simulink model "mcb_host_model_f28069m"  (R2025b)
settings: Solver=FixedStepDiscrete  StartTime=0.0  StopTime=inf  RelTol=1e-3  EnableMultiTasking=on
values from neighbouring files (symbols this model uses):
  PU_System = mcb.getPUSystemParameters(bldc,inverter)    [mcb_bldc_sixstep_f28069mLaunchPad_data.m]    (also in mcb_bldc_sixstep_f28379d_data.m = mcb.getPUSystemParameters(bldc, inverter))
  Ts = T_pwm    (= 5e-05)    [mcb_bldc_sixstep_f28069mLaunchPad_data.m]    (also in mcb_bldc_sixstep_f28379d_data.m = 3e-05)
libraries: instrumentseriallib x3
settings Model: Creator=The MathWorks, Inc.  LastModifiedBy=The MathWorks, Inc.
settings SolverCC: AlgebraicLoopSolver=TrustRegion  MaxZcPerStep=1.0
settings DataIOCC: LimitDataPoints=on  SaveFormat=Array  ReturnWorkspaceOutputs=off
settings OptimizationCC: ReuseModelBlockBuffer=off  LifeSpan=1  EfficientTunableParamExpr=on
settings DebuggingCC: UnderspecifiedInitializationDetection=Classic  MergeDetectMultiDrivingBlocksExec=none  SolverPrmCheckMsg=warning  ParameterPrecisionLossMsg=none  UnconnectedInputMsg=warning  UnconnectedOutputMsg=warning  UnconnectedLineMsg=warning  AllowSymbolicDim=off  PregeneratedLibrarySubsystemCodeDiagnostic=none  SFUnexpectedBacktrackingDiag=warning  SFNoUnconditionalDefaultTransitionDiag=warning  SFExecutionAtInitializationDiag=none  ArithmeticOperatorsInVariantConditions=warning
settings HardwareCC: ProdBitPerPointer=32.0  ProdLargestAtomicFloat=None  ProdIntDivRoundTo=Undefined  ProdEndianess=Unspecified  ProdWordSize=32.0  ProdHWDeviceType=32-bit Generic
settings ModelReferenceCC: EnableRefExpFcnMdlSchedulingChecks=on  PropagateSignalLabelsOutOfModel=off
settings SFSimCC: SimUseLocalCustomCode=off  MATLABDynamicMemAlloc=off
settings RTWCC: SystemTargetFile=ert.tlc  TemplateMakefile=ert_default_tmf  GenerateReport=on  RTWUseLocalCustomCode=off  IncludeHyperlinkInReport=on  LaunchReport=on  GenerateTraceInfo=on  GenerateTraceReport=on  GenerateTraceReportSl=on  GenerateTraceReportSf=on  GenerateTraceReportEml=on  GPUComputeCapability=3.5  DLArmComputeVersion=19.05  Description=Real-Time Workshop Embedded Coder
settings CodeAppCC: IgnoreCustomStorageClasses=off  StateflowObjectComments=on  InternalIdentifier=Classic
settings ERTTargetCC: InlinedParameterPlacement=Hierarchical  ERTCustomFileTemplate=example_file_process.tlc  ConvertIfToSwitch=off  SuppressUnreachableDefaultCases=off  DynamicArrayContainerType=coder::array  MultiwordLength=2048.0  GenerateSampleERTMain=on
settings ConfigComp: CovMetricSettings=dw  CovSaveCumulativeToWorkspaceVar=on  CovSaveSingleToWorkspaceVar=on  CovExternalEMLEnable=off  CovSFcnEnable=off

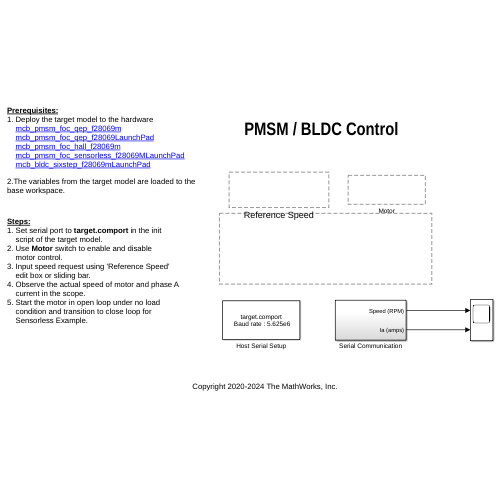
[thumbnail: Simulink's stored preview of the top-level diagram]
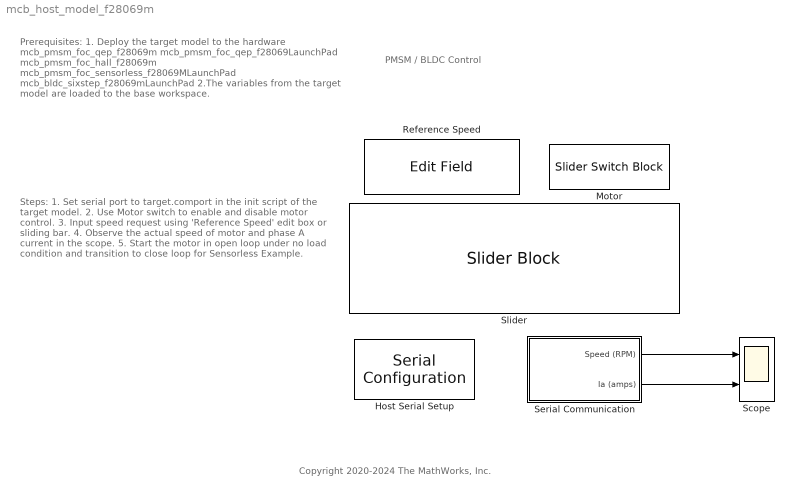
== system mcb_host_model_f28069m ==
  note: Copyright 2020-2024 The MathWorks, Inc.
  note: Steps:
      | 1. Set serial port to target.comport in the init
      | script of the target model.
      | 2. Use Motor switch to enable and disable
      | motor control.
      | 3. Input speed request using 'Reference Speed'
      | edit box or sliding bar.
      | 4. Observe the actual speed of motor and phase A
      | current in the scope.
      | 5. Start the motor in open loop under no load
      | condition and transition to close loop for
      | Sensorless Example.
  note: PMSM / BLDC Control
  note: Prerequisites:
      | 1. Deploy the target model to the hardware
      | mcb_pmsm_foc_qep_f28069m
      | mcb_pmsm_foc_qep_f28069LaunchPad
      | mcb_pmsm_foc_hall_f28069m
      | mcb_pmsm_foc_sensorless_f28069MLaunchPad
      | mcb_bldc_sixstep_f28069mLaunchPad
      |
      | 2.The variables from the target model are loaded to the base workspace.
  Host Serial Setup : instrumentseriallib/Serial Configuration  Priority=-99  PortSel=target.comport  Port=target.comport  ComPort=target.comport  BaudRate=5.625e6  DataBits=8  Parity=none  StopBits=1  ByteOrder=little-endian  FlowControl=none  Timeout=2  SimulateUsing=Interpreted execution  BlockInModel=on  aMode=5
      settings: LibrarySourceBlock=mcblib/Protection and Diagnostics/Host Serial Setup
  Motor : SliderSwitchBlock  LabelPosition=Hide
  Reference Speed : EditField  LabelPosition=Hide  ShowInitialText=on  Alignment=Center
  Scope : Scope  NumInputPorts=2
      settings: Title=Speed  ActiveDisplayYMinimum=-6000  ActiveDisplayYMaximum=6000  YLabel=Speed (RPM)
  Serial Communication : Subsystem
  Slider : SliderBlock  LabelPosition=Hide  ScaleMin=-6000  ScaleMax=6000
  wires:
  Serial Communication/1(Speed (RPM)) -> Scope/1
  Serial Communication/2(Ia (amps)) -> Scope/2

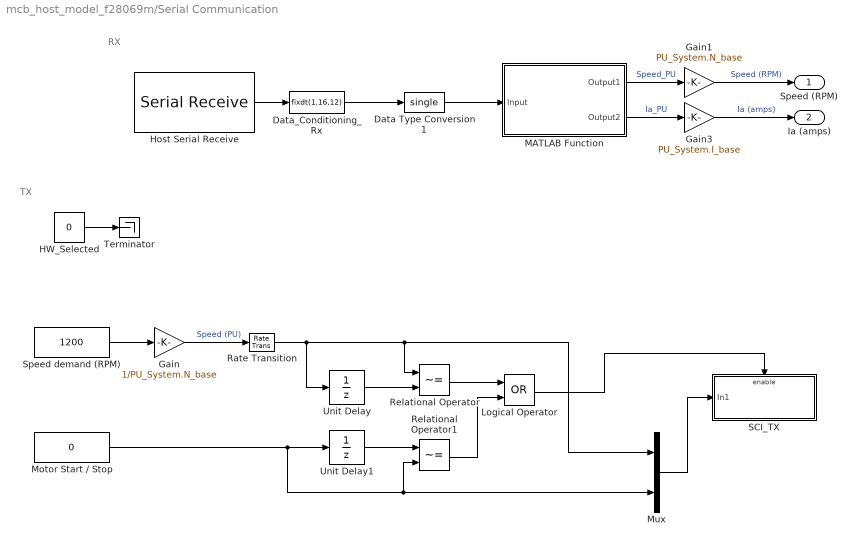
== system mcb_host_model_f28069m/Serial Communication ==
  note: RX
  note: TX
  Data Type Conversion1 : DataTypeConversion  OutDataTypeStr=single  RndMeth=Simplest  SaturateOnIntegerOverflow=off
  Data_Conditioning_Rx : DataTypeConversion  OutDataTypeStr=fixdt(1,16,12)  ConvertRealWorld=Stored Integer (SI)  RndMeth=Simplest  SaturateOnIntegerOverflow=off
  Gain : Gain  Gain=1/PU_System.N_base  RndMeth=Simplest  OutDataTypeStr=Inherit: Same as input
  Gain1 : Gain  Gain=PU_System.N_base  OutDataTypeStr=single  RndMeth=Simplest
  Gain3 : Gain  Gain=PU_System.I_base  OutDataTypeStr=single  RndMeth=Simplest
  HW_Selected : Constant  Value=0  OutDataTypeStr=uint8
  Host Serial Receive : instrumentseriallib/Serial Receive  PortSel=target.comport  Port=target.comport  ComPort=target.comport  DataType=uint16  SaveDataType=uint8  ToggleHeader=on  Header='SS'  ToggleDataSize=on  DataSize=[600 2]  ToggleTerminator=on  Terminator=Custom terminator  CustomTerminator='EE'  InputFormat=Row major  EnableBlockingMode=on  ActionDataUnavailable=Output last received value  ActionWhenDataUnavailable=Output last received value  CustomValue=0  SampleTime=600 * Ts  SimulateUsing=Interpreted execution  BlockInModel=on  aMode=5  LibraryInUse=instrumentlib
      settings: LibrarySourceBlock=mcblib/Protection and Diagnostics/Host Serial Receive
  Logical Operator : Logic  Operator=OR  AllPortsSameDT=off  OutDataTypeStr=boolean
  MATLAB Function : MATLAB Function  TreatAsAtomicUnit=on
  Motor Start / Stop : Constant  Value=0  VectorParams1D=off  OutDataTypeStr=single  SampleTime=0.03
  Mux : Mux  Inputs=2
  Rate Transition : RateTransition  OutPortSampleTime=0.03
  Relational Operator : RelationalOperator  Operator=~=  OutDataTypeStr=boolean  InputSameDT=off
  Relational Operator1 : RelationalOperator  Operator=~=  OutDataTypeStr=boolean  InputSameDT=off
  SCI_TX : Subsystem  TreatAsAtomicUnit=on
  Speed demand (RPM) : Constant  Value=1200  VectorParams1D=off  OutDataTypeStr=single  SampleTime=0.03
  Terminator : Terminator
  Unit Delay : UnitDelay  InitialCondition=0.5  SampleTime=-1  HasFrameUpgradeWarning=on
  Unit Delay1 : UnitDelay  SampleTime=-1  HasFrameUpgradeWarning=on
  Speed (RPM) : Outport
  Ia (amps) : Outport  Port=2
  wires:
  HW_Selected/1 -> Terminator/1
  Unit Delay1/1 -> Relational Operator1/1
  Relational Operator1/1 -> Logical Operator/2
  Unit Delay/1 -> Relational Operator/2
  Relational Operator/1 -> Logical Operator/1
  Gain/1 -> Rate Transition/1  "Speed (PU)"
  Speed demand (RPM)/1 -> Gain/1
  Mux/1 -> SCI_TX/1(In1)
  Rate Transition/1 -> Unit Delay/1, Mux/1, Relational Operator/1
  Logical Operator/1 -> SCI_TX/Enable
  Motor Start / Stop/1 -> Relational Operator1/2, Mux/2, Unit Delay1/1
  MATLAB Function/2(Output2) -> Gain3/1  "Ia_PU"
  Gain3/1 -> Ia (amps)/1  "Ia (amps)"
  Host Serial Receive/1 -> Data_Conditioning_Rx/1
  MATLAB Function/1(Output1) -> Gain1/1  "Speed_PU"
  Gain1/1 -> Speed (RPM)/1  "Speed (RPM)"
  Data_Conditioning_Rx/1 -> Data Type Conversion1/1
  Data Type Conversion1/1 -> MATLAB Function/1(Input)

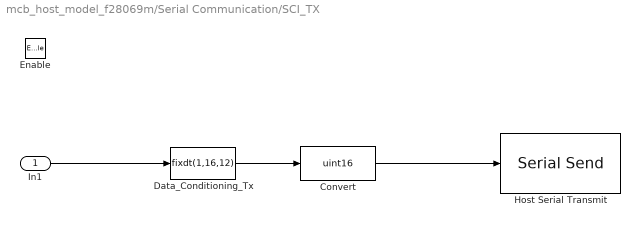
== system mcb_host_model_f28069m/Serial Communication/SCI_TX ==
  In1 : Inport
  Enable : EnablePort
  Convert : DataTypeConversion  OutDataTypeStr=uint16  ConvertRealWorld=Stored Integer (SI)  RndMeth=Simplest  SaturateOnIntegerOverflow=off
  Data_Conditioning_Tx : DataTypeConversion  OutDataTypeStr=fixdt(1,16,12)  RndMeth=Simplest  SaturateOnIntegerOverflow=off
  Host Serial Transmit : instrumentseriallib/Serial Send  PortSel=target.comport  Port=target.comport  ComPort=target.comport  Header=[]  Terminator=<none>  CustomTerminator=[]  EnableBlockingMode=off  SimulateUsing=Interpreted execution  BlockInModel=on  aMode=5
      settings: LibrarySourceBlock=mcblib/Protection and Diagnostics/Host Serial Transmit
  wires:
  Convert/1 -> Host Serial Transmit/1
  Data_Conditioning_Tx/1 -> Convert/1
  In1/1 -> Data_Conditioning_Tx/1

== matlab function mcb_host_model_f28069m/Serial Communication/MATLAB Function ==
  data: Output1 output; Output2 output; Input input
function [ Output1, Output2] = unBuf(Input)

Output1 = Input(:, 1);
Output2 = Input(:, 2);
end
